simulink model "circuit_with_initial_motor_model"  (R2024b)
settings: Solver=VariableStepAuto  StartTime=0  StopTime=0.5  FixedStep=1e-6  RelTol=1e-3
libraries: spsDiodeLib x6, spsMeanLib x4, spsMosfetLib x4, spsACVoltageSourceLib x3, spsCurrentMeasurementLib x3, spsParallelRLCBranchLib x3, spsSeriesRLCBranchLib x3, spsVoltageMeasurementLib x3, spsDCMachineLib x1, spsDCVoltageSourceLib x1, spsGroundLib x1, spsRMSLib x1
settings Model: Creator=06MBC93  LastModifiedBy=kamer
settings RTWCC: GPUComputeCapability=3.5

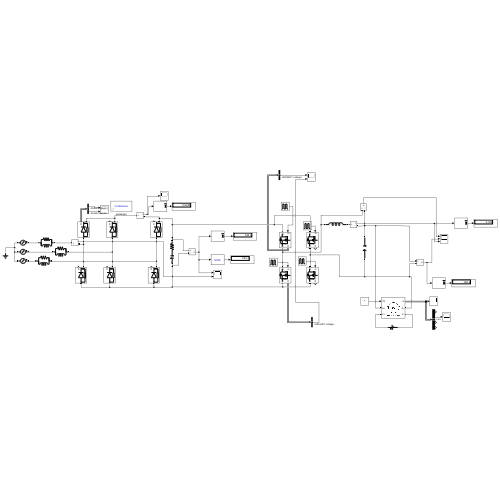
[thumbnail: Simulink's stored preview of the top-level diagram]
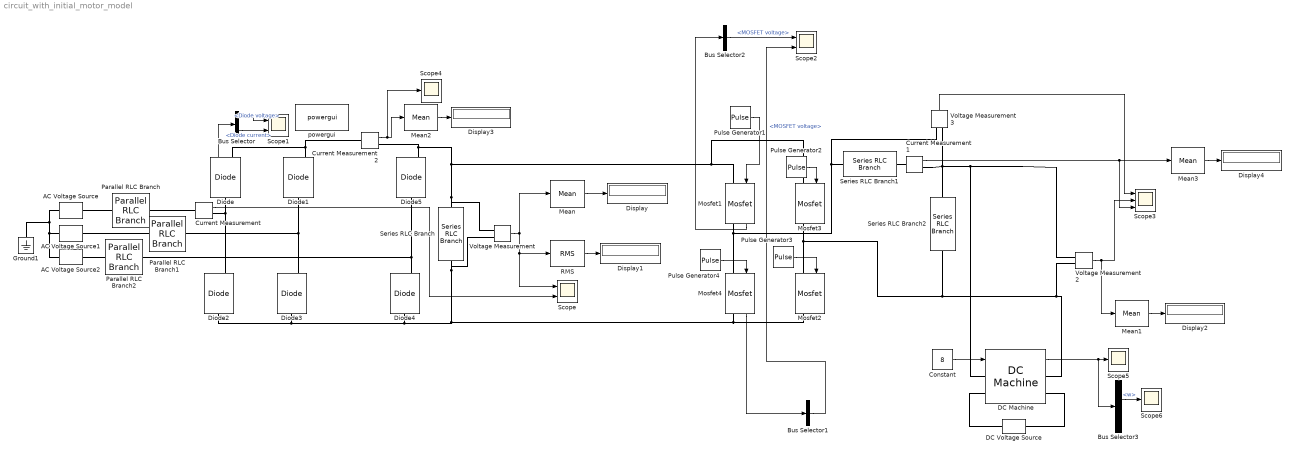
== system circuit_with_initial_motor_model ==
  AC Voltage Source : spsACVoltageSourceLib/AC Voltage Source  Amplitude=325  Phase=0  Frequency=50  SampleTime=0  Measurements=None  BusType=swing  Pref=10e3  Qref=0  Qmin=-inf  Qmax=+inf
  AC Voltage Source1 : spsACVoltageSourceLib/AC Voltage Source  Amplitude=325  Phase=120  Frequency=50  SampleTime=0  Measurements=None  BusType=swing  Pref=10e3  Qref=0  Qmin=-inf  Qmax=+inf
  AC Voltage Source2 : spsACVoltageSourceLib/AC Voltage Source  Amplitude=325  Phase=240  Frequency=50  SampleTime=0  Measurements=None  BusType=swing  Pref=10e3  Qref=0  Qmin=-inf  Qmax=+inf
  Bus Selector : BusSelector  OutputSignals=Diode voltage,Diode current
  Bus Selector1 : BusSelector  OutputSignals=MOSFET voltage
  Bus Selector2 : BusSelector  OutputSignals=MOSFET voltage
  Bus Selector3 : BusSelector  OutputSignals=Te,w,iF,iA
  Constant : Constant  Value=8
  Current Measurement : spsCurrentMeasurementLib/Current Measurement  PhasorSimulation=off  OutputType=Complex  PSBequivalent=0
  Current Measurement1 : spsCurrentMeasurementLib/Current Measurement  PhasorSimulation=off  OutputType=Complex  PSBequivalent=0
  Current Measurement2 : spsCurrentMeasurementLib/Current Measurement  PhasorSimulation=off  OutputType=Complex  PSBequivalent=0
  DC Machine : spsDCMachineLib/DC Machine  PresetModel=No  MechanicalLoad=Torque TL  FieldType=Wound  ShowDetailedParameters=on  MeasurementBus=on  RLa="[ 0.8  0.0125]"  RLf="[ 210  23]"  Laf=1.8  MachineConstant=Torque constant (N.m/A)  Ke=1.8  Kt=1.8  J=0.1  Bm=0  Tf=0.2  w0=1  Ifinit=1.04761904756944  TsPowergui=0  TsBlock=-1
  DC Voltage Source : spsDCVoltageSourceLib/DC Voltage Source  Amplitude=220  Measurements=None
  Diode{,1..5} (6 alike) : spsDiodeLib/Diode  Ron=0.001  Lon=0  Vf=0.8  IC=0  UseSnubber=0  Rs=5000  Cs=250e-9  Measurements=on
  Display{,1..4} (5 alike) : Display
  Ground1 : spsGroundLib/Ground  LConnTagsString=a
  Mean : spsMeanLib/Mean  Freq=300  Vinit=0  Ts=0
  Mean1 : spsMeanLib/Mean  Freq=60  Vinit=0  Ts=0
  Mean2 : spsMeanLib/Mean  Freq=60  Vinit=0  Ts=0
  Mean3 : spsMeanLib/Mean  Freq=60  Vinit=0  Ts=0
  Mosfet{1..4} (4 alike) : spsMosfetLib/Mosfet  Ron=0.1  Lon=0  Rd=0.01  Vfd=0  IC=0  Rs=1e5  Cs=inf  Measurements=on
  Parallel RLC Branch : spsParallelRLCBranchLib/Parallel RLC Branch  LConnTagsString=a  RConnTagsString=__new0  BranchType=RL  Resistance=1e+4  Inductance=1e-2  SetiL0=off  InitialCurrent=0  Capacitance=1e-6  Setx0=off  InitialVoltage=0  Measurements=None
  Parallel RLC Branch1 : spsParallelRLCBranchLib/Parallel RLC Branch  LConnTagsString=a  RConnTagsString=__new0  BranchType=RL  Resistance=1e+4  Inductance=1e-2  SetiL0=off  InitialCurrent=0  Capacitance=1e-6  Setx0=off  InitialVoltage=0  Measurements=None
  Parallel RLC Branch2 : spsParallelRLCBranchLib/Parallel RLC Branch  LConnTagsString=a  RConnTagsString=__new0  BranchType=RL  Resistance=1e+4  Inductance=1e-2  SetiL0=off  InitialCurrent=0  Capacitance=1e-6  Setx0=off  InitialVoltage=0  Measurements=None
  Pulse Generator1 : DiscretePulseGenerator  PulseType=Time based  Amplitude=10  Period=1/25000  PulseWidth=35
  Pulse Generator2 : DiscretePulseGenerator  PulseType=Time based  Amplitude=0  Period=1/25000  PulseWidth=35  PhaseDelay=1/50000
  Pulse Generator3 : DiscretePulseGenerator  PulseType=Time based  Amplitude=10  Period=1/25000  PulseWidth=99.99
  Pulse Generator4 : DiscretePulseGenerator  PulseType=Time based  Amplitude=10  Period=1/25000  PulseWidth=65  PhaseDelay=35/2500000
  RMS : spsRMSLib/RMS  TrueRMS=on  Freq=300  RMSInit=0  Ts=0
  Scope : Scope  NumInputPorts=2
  Scope1 : Scope  NumInputPorts=2
  Scope2 : Scope  NumInputPorts=2
  Scope3 : Scope  NumInputPorts=3
  Scope4 : Scope
  Scope5 : Scope
  Scope6 : Scope
  Series RLC Branch : spsSeriesRLCBranchLib/Series RLC Branch  LConnTagsString=__new0  RConnTagsString=__new0  BranchType=RC  Resistance=1e-6  Inductance=1e-3  SetiL0=off  InitialCurrent=0  Capacitance=1e-6  Setx0=off  InitialVoltage=0  Measurements=None
  Series RLC Branch1 : spsSeriesRLCBranchLib/Series RLC Branch  LConnTagsString=__new0  RConnTagsString=__new0  BranchType=L  Resistance=1  Inductance=3e-3  SetiL0=off  InitialCurrent=0  Capacitance=1e-6  Setx0=off  InitialVoltage=0  Measurements=None
  Series RLC Branch2 : spsSeriesRLCBranchLib/Series RLC Branch  LConnTagsString=__new0  RConnTagsString=__new0  BranchType=C  Resistance=1  Inductance=1e-3  SetiL0=off  InitialCurrent=0  Capacitance=3e-6  Setx0=off  InitialVoltage=0  Measurements=None
  Voltage Measurement : spsVoltageMeasurementLib/Voltage Measurement  PhasorSimulation=off  OutputType=Complex  PSBequivalent=0
  Voltage Measurement2 : spsVoltageMeasurementLib/Voltage Measurement  PhasorSimulation=off  OutputType=Complex  PSBequivalent=0
  Voltage Measurement3 : spsVoltageMeasurementLib/Voltage Measurement  PhasorSimulation=off  OutputType=Complex  PSBequivalent=0
  powergui : sps_lib/powergui  Priority=1  SimulationMode=Continuous  SampleTime=50e-6  frequency=60  Iterations=50  frequencyindice=50  Pbase=100e6  ErrMax=1e-4  UnitsV=kV  UnitsW=MW  buscounter=0  FunctionMessages=off  echomessages=off  EnableUseOfTLC=off  CurrentSourceSwitches=off  DisableSnubberDevices=off  DisableRonSwitches=off  DisableVfSwitches=off  DisplayEquations=off  AutomaticDiscreteSolvers=off  SolverType=Tustin/Backward Euler (TBE)  Interpol=off  ExternalGateDelay=off  methode=off  Ts=100  x0status=blocks  SPID=on  SwTol=0  HookPort=off  NonlinearTolerance=1e-4  nMaxIteration=100  ContinueOnMaxIteration=off  RestoreLinks=warning  ResistiveCurrentMeasurement=off  Frange=[0:2:500]  Ylog=off  Xlog=on  ShowGrid=off  save=off  variable=ZData  structure=0  ZoomFFT=off  StartTime=0.0  cycles=1  DisplayStyle=1  fundamental=60  FreqAxis=off  MaxFrequency=1000  frequencyindicesteady=1  RmsSteady=1  display=off
  wires:
  Mean/1 -> Display/1
  Voltage Measurement/1 -> Mean/1, Scope/1, RMS/1
  Current Measurement/1 -> Scope/2
  RMS/1 -> Display1/1
  Diode/1 -> Bus Selector/1
  Bus Selector/2 -> Scope1/2  "<Diode current>"
  Bus Selector/1 -> Scope1/1  "<Diode voltage>"
  Voltage Measurement3/1 -> Scope3/1
  Voltage Measurement2/1 -> Mean1/1, Scope3/2
  Current Measurement1/1 -> Mean3/1, Scope3/3
  Mean1/1 -> Display2/1
  Current Measurement2/1 -> Scope4/1, Mean2/1
  Mean2/1 -> Display3/1
  Mean3/1 -> Display4/1
  Pulse Generator1/1 -> Mosfet1/1
  Pulse Generator3/1 -> Mosfet2/1
  Pulse Generator2/1 -> Mosfet3/1
  Pulse Generator4/1 -> Mosfet4/1
  Bus Selector1/1 -> Scope2/2  "<MOSFET voltage>"
  Bus Selector2/1 -> Scope2/1  "<MOSFET voltage>"
  Mosfet4/1 -> Bus Selector1/1
  Mosfet1/1 -> Bus Selector2/1
  DC Machine/1 -> Bus Selector3/1, Scope5/1
  Bus Selector3/2 -> Scope6/1  "<w>"
  Constant/1 -> DC Machine/1
  connections:
  AC Voltage Source/LConn1 -- Ground1/LConn1 -- AC Voltage Source2/LConn1 -- AC Voltage Source1/LConn1
  Diode2/RConn1 -- Current Measurement/RConn1 -- Diode/LConn1
  Diode3/RConn1 -- Parallel RLC Branch1/RConn1 -- Diode1/LConn1
  Diode4/RConn1 -- Parallel RLC Branch2/RConn1 -- Diode5/LConn1
  Voltage Measurement/LConn1 -- Series RLC Branch/LConn1 -- Mosfet1/LConn1 -- Mosfet3/LConn1 -- Current Measurement2/RConn1 -- Diode5/RConn1
  Diode2/LConn1 -- Diode3/LConn1 -- Mosfet4/RConn1 -- Mosfet2/RConn1 -- Voltage Measurement/LConn2 -- Series RLC Branch/RConn1 -- Diode4/LConn1
  Series RLC Branch1/RConn1 -- Current Measurement1/LConn1
  Parallel RLC Branch/RConn1 -- Current Measurement/LConn1
  Diode/RConn1 -- Diode1/RConn1 -- Current Measurement2/LConn1
  AC Voltage Source/RConn1 -- Parallel RLC Branch/LConn1
  AC Voltage Source1/RConn1 -- Parallel RLC Branch1/LConn1
  AC Voltage Source2/RConn1 -- Parallel RLC Branch2/LConn1
  Mosfet2/LConn1 -- Voltage Measurement2/LConn2 -- DC Machine/RConn1 -- Series RLC Branch2/RConn1 -- Mosfet3/RConn1
  DC Voltage Source/LConn1 -- DC Machine/RConn2
  DC Machine/LConn2 -- DC Voltage Source/RConn1
  Mosfet1/RConn1 -- Voltage Measurement3/LConn1 -- Series RLC Branch1/LConn1 -- Mosfet4/LConn1
  Voltage Measurement2/LConn1 -- DC Machine/LConn1 -- Voltage Measurement3/LConn2 -- Current Measurement1/RConn1 -- Series RLC Branch2/LConn1
